simulink model "sampleModel1488"  (R2023a)
settings: Solver=VariableStepAuto  StartTime=0.0  StopTime=10.0  RelTol=1e-3
undefined symbols (not defined in the file): b011101a, b0c8, bf87616c, DiscIntNeverNeededParam, Newton, Raphson
libraries: simulink x171, slpidlib x32, simulink_need_slupdate x2
(part 1 of 6)
settings Model: Creator=TSMC  LastModifiedBy=TSMC

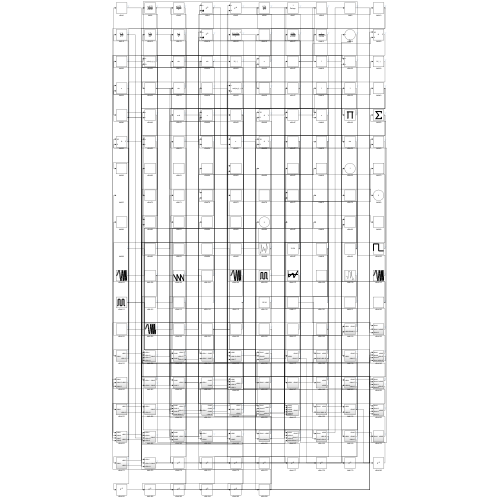
[thumbnail: Simulink's stored preview of the top-level diagram]
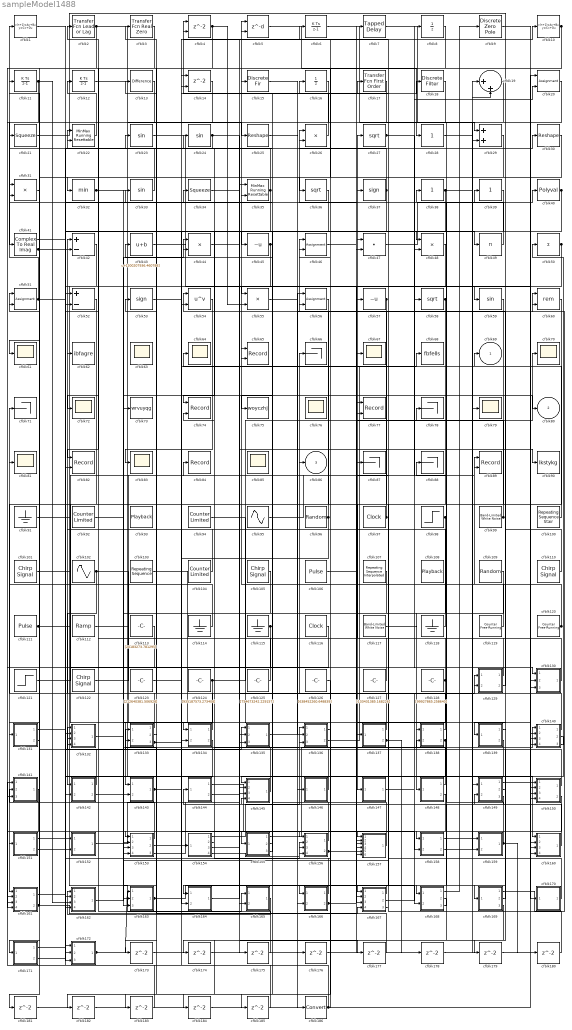
== system sampleModel1488 ==
  cfblk1 : DiscreteStateSpace
  cfblk10 : DiscreteStateSpace
  cfblk100 : simulink/Sources/Repeating Sequence Stair  OutValues=[-762369518.443559, -847374089.038324]  tsamp=-1  OutMin=[]  OutMax=[]  OutDataTypeStr=double  OutputDataTypeScalingMode=double  OutDataType=fixdt(0,8)  ConRadixGroup=Best Precision: Vector-wise  OutScaling=2^-12
  cfblk101 : simulink/Sources/Chirp Signal  f1=[899816213.693097]  T=[-380286117.262630]  f2=[198637424.557367]
  cfblk102 : Sin  Amplitude=[-477515735.570016]  Bias=[72041173.991796]  SampleTime=0
  cfblk103 : simulink/Sources/Repeating Sequence  rep_seq_t=[0 2]  rep_seq_y=[-391359167.323341, -994559578.240211]
  cfblk104 : simulink/Sources/Counter Limited  uplimit=[518.000000]  tsamp=-1
  cfblk105 : simulink/Sources/Chirp Signal  f1=[828543943.259845]  T=[-687971089.943261]  f2=[529515713.712588]
  cfblk106 : DiscretePulseGenerator  PulseType=Time based  Amplitude=[720280650.254154]  Period=[58198645.361039]  PulseWidth=5  PhaseDelay=[7.000000]
  cfblk107 : simulink/Sources/Repeating Sequence Interpolated  OutValues=[129302697.254445, -483455900.765630, 289136432.217906, -604021489.155862, 732674675.731693]  TimeValues=[0 0.1 0.5 0.6 1].'  LookUpMeth=Use Input Below  tsamp=0.01  OutMin=[]  OutMax=[]  OutDataTypeStr=double  OutputDataTypeScalingMode=double  OutDataType=fixdt(0,8)  OutScaling=2^-10
  cfblk108 : Playback  NumPorts=0  PartName=b011101a-6eb5-4819-b0c8-95222edf8c13
  cfblk109 : RandomNumber  Mean=[-63804.166528]  Variance=[5878.142676]  Seed=[575719339.000000]  SampleTime=0.1
  cfblk11 : DiscreteIntegrator  ICPrevOutput=DiscIntNeverNeededParam  ICPrevScaledInput=DiscIntNeverNeededParam
  cfblk110 : simulink/Sources/Chirp Signal  f1=[-302225759.290162]  T=[865618805.379564]  f2=[-592318645.179689]
  cfblk111 : DiscretePulseGenerator  PulseType=Time based  Amplitude=[753444769.039848]  Period=[70377866.971397]  PulseWidth=5  PhaseDelay=[4.000000]
  cfblk112 : simulink/Sources/Ramp  slope=[-695.666721]  start=[46.584433]  InitialOutput=[-395183.012407]
  cfblk113 : Constant  Value=[20183273.781295]  SampleTime=1
  cfblk{91,114..115,118} (4 alike) : Ground
  cfblk116 : DigitalClock
  cfblk117 : simulink/Sources/Band-Limited White Noise  Cov=[1552995708.106671]  Ts=0.1  seed=[2294206463.000000]
  cfblk119 : simulink/Sources/Counter Free-Running  NumBits=[2.000000]  tsamp=-1
  cfblk12 : DiscreteIntegrator  ICPrevOutput=DiscIntNeverNeededParam  ICPrevScaledInput=DiscIntNeverNeededParam
  cfblk120 : simulink/Sources/Counter Free-Running  NumBits=[18.000000]  tsamp=-1
  cfblk121 : Step  Time=[19.000000]  Before=[420474009.001986]  After=[851009496.390192]  SampleTime=0
  cfblk122 : simulink/Sources/Chirp Signal  f1=[-178285749.618264]  T=[-856050795.136190]  f2=[-767698347.330060]
  cfblk123 : Constant  Value=[212640381.506928]  SampleTime=1
  cfblk124 : Constant  Value=[935187573.273408]  SampleTime=1
  cfblk125 : Constant  Value=[754673242.229157]  SampleTime=1
  cfblk126 : Constant  Value=[638452260.648839]  SampleTime=1
  cfblk127 : Constant  Value=[133431385.168226]  SampleTime=1
  cfblk128 : Constant  Value=[99927865.258640]  SampleTime=1
  cfblk129 : Subsystem
  cfblk13 : simulink/Discrete/Difference  ICPrevInput=0.0  OutMin=[]  OutMax=[]  OutDataTypeStr=Inherit: Inherit via back propagation  OutDataType=fixdt(1, 16)  OutScaling=2^-10  DoSatur=off
  cfblk130 : Subsystem
  cfblk131 : Subsystem
  cfblk132 : Subsystem
  cfblk133 : Subsystem
  cfblk134 : Subsystem
  cfblk135 : Subsystem
  cfblk136 : Subsystem
  cfblk137 : Subsystem
  cfblk138 : Subsystem
  cfblk139 : Subsystem
  cfblk14 : Delay  ShowEnablePort=on  SampleTime=1
      settings: InputPortMap=u0,e6
  cfblk140 : Subsystem
  cfblk141 : Subsystem
  cfblk142 : Subsystem
  cfblk143 : Subsystem
  cfblk144 : Subsystem
  cfblk145 : Subsystem
  cfblk146 : Subsystem
  cfblk147 : Subsystem
  cfblk148 : Subsystem
  cfblk149 : Subsystem
  cfblk15 : DiscreteFir  SampleTime=1
  cfblk150 : Subsystem
  cfblk151 : Subsystem
  cfblk152 : Subsystem
  cfblk153 : Subsystem
  cfblk154 : Subsystem
  cfblk155 : Subsystem
  cfblk156 : Subsystem
  cfblk157 : Subsystem
  cfblk158 : Subsystem
  cfblk159 : Subsystem
  cfblk16 : UnitDelay  HasFrameUpgradeWarning=on
  cfblk160 : Subsystem
  cfblk161 : Subsystem
  cfblk162 : Subsystem
  cfblk163 : Subsystem
  cfblk164 : Subsystem
  cfblk165 : Subsystem
  cfblk166 : Subsystem
  cfblk167 : Subsystem
  cfblk168 : Subsystem
  cfblk169 : Subsystem
  cfblk17 : simulink/Discrete/Transfer Fcn First Order  PoleZ=0.95  ICPrevOutput=0.0  DoSatur=off
  cfblk170 : Subsystem
  cfblk171 : Subsystem
  cfblk172 : Subsystem
  cfblk{173..185} (13 alike) : Delay  SampleTime=1
  cfblk18 : DiscreteFilter  SampleTime=1
  cfblk186 : DataTypeConversion  SaturateOnIntegerOverflow=off  RndMeth=Floor
  cfblk19 : Sum  Inputs=|++
  cfblk2 : simulink/Discrete/Transfer Fcn Lead or Lag  PoleZ=0.95  ZeroZ=0.75  ICPrevOutput=0.0  ICPrevInput=0.0  DoSatur=off
  cfblk{20,46,51,56} (4 alike) : Assignment  DiagnosticForDimensions=Warning  IndexOptions=Index vector (dialog)  Indices=1  OutputSizes=1
  cfblk21 : Squeeze
  cfblk22 : simulink/Math Operations/MinMax Running Resettable  Function=min  vinit=0.0
  cfblk{23..24,33,59} (4 alike) : Trigonometry
  cfblk25 : Reshape
  cfblk{26,44,48,55} (4 alike) : Product  Inputs=**
  cfblk27 : Sqrt
  cfblk28 : simulink/Math Operations/Slider Gain  gain=1  low=0  high=2
  cfblk29 : Sum
  cfblk3 : simulink/Discrete/Transfer Fcn Real Zero  ZeroZ=0.75  ICPrevInput=0.0  DoSatur=off
  cfblk30 : Reshape
  cfblk31 : Product
  cfblk32 : MinMax
  cfblk34 : Squeeze
  cfblk35 : simulink/Math Operations/MinMax Running Resettable  Function=min  vinit=0.0
  cfblk36 : Sqrt
  cfblk37 : Signum
  cfblk38 : simulink/Math Operations/Slider Gain  gain=1  low=0  high=2
  cfblk39 : simulink/Math Operations/Slider Gain  gain=1  low=0  high=2
  cfblk4 : Delay  ShowEnablePort=on  SampleTime=1
      settings: InputPortMap=u0,e6
  cfblk40 : Polyval  Coefs=[ +2.081618890e-019, -1.441693666e-014, +4.719686976e-010, -8.536869453e-006, +1.621573104e-001, -8.087801117e+001 ]
  cfblk41 : ComplexToRealImag
  cfblk42 : Sum  Inputs=+-
  cfblk43 : Bias  Bias=[200207936.460788]  SaturateOnIntegerOverflow=off
  cfblk45 : UnaryMinus
  cfblk47 : DotProduct  OutDataTypeStr=Inherit: Inherit via internal rule
  cfblk49 : Product  Inputs=*
  cfblk5 : Delay  DelayLengthSource=Input port  SampleTime=1
      settings: InputPortMap=u0,p1
  cfblk50 : Sum  Inputs=+
  cfblk52 : Sum  Inputs=+-
  cfblk53 : Signum
  cfblk54 : Math  Operator=pow
  cfblk57 : UnaryMinus
  cfblk58 : Sqrt
  cfblk6 : DiscreteIntegrator  ICPrevOutput=DiscIntNeverNeededParam  ICPrevScaledInput=DiscIntNeverNeededParam
  cfblk60 : Math  Operator=rem
  cfblk{61,63..64,67,70,72,76,79,81,83,85} (11 alike) : Scope
      cfblk63 settings: Floating=on
      cfblk76 settings: Floating=on
      cfblk85 settings: Floating=on
  cfblk62 : ToWorkspace  VariableName=ibfagre  SaveFormat=Timeseries  SampleTime=-1
  cfblk65 : Record  FileSettingsInternal="{\"entries\":[{\"content\":{\"excelSettings\":{\"content\":{},\"type\":\"Streamout.ExcelSettings\"}},\"type\":\"Streamout.FileSettingStorage\",\"uuid\":\"\"}],\"packageUris\":[\"http:\\/\\/schema.mathworks.com\\/mf0\\/streamout_blocks\\/R2020a\"],\"version\":\"1.0\"}"  Layout=[1 1]  SignalsInternal="{\"entries\":[{\"content\":{\"signals\":[{\"content\":{\"blockPath\":[],\"dimensions\":[1],\"domain\":\"\",\"lineColor\":\"#a2142f\",\"plots\":[1],\"port\":1,\"sid\":[\"\"],\"signalID\":13705,\"signalName\":\"cfblk143\"},\"type\":\"RecordBlkView.Signal\",\"uuid\":\"\"},{\"content\":{\"blockPath\":[],\"dimensions\":[1],\"domain\":\"\",\"lineColor\":\"#139fff\",\"plots\":[1],\"port\":2,\"sid\":[\"\"],\"signalID\":13793,\"signalName\":\"cfblk115\"},\"type\":\"RecordBlkView.Signal\",\"uuid\":\"\"}]},\"type\":\"RecordBlkView.InputSignals\",\"uuid\":\"\"}],\"packageUris\":[\"http:\\/\\/schema.mathworks.com\\/mf0\\/streamout_blocks\\/R2020a\"],\"version\":\"1.0\"}"  VisualizationBindings="{\"xyplotplugin\":{\"info\":[{\"series\":[{\"bindingParametersList\":[{\"parameter\":\"X-Axis\",\"signalID\":13705,\"signalName\":\"cfblk143\"},{\"parameter\":\"Y-Axis\",\"signalID\":13793,\"signalName\":\"cfblk115\"}],\"seriesID\":56317}],\"subplotID\":1}]}}"  CompatibilityTag=XY
  cfblk{66,71,78,87..88} (5 alike) : Terminator
  cfblk68 : ToWorkspace  VariableName=fbfells  SaveFormat=Timeseries  SampleTime=-1
  cfblk7 : simulink/Discrete/Tapped Delay  vinit=0.0  samptime=-1  NumDelays=1  DelayOrder=Oldest  includeCurrent=off
  cfblk73 : ToWorkspace  VariableName=wrvuyqg  SaveFormat=Timeseries  SampleTime=-1
  cfblk74 : Record  FileSettingsInternal="{\"entries\":[{\"content\":{\"excelSettings\":{\"content\":{},\"type\":\"Streamout.ExcelSettings\"}},\"type\":\"Streamout.FileSettingStorage\",\"uuid\":\"\"}],\"packageUris\":[\"http:\\/\\/schema.mathworks.com\\/mf0\\/streamout_blocks\\/R2020a\"],\"version\":\"1.0\"}"  Layout=[1 1]  SignalsInternal="{\"entries\":[{\"content\":{\"signals\":[{\"content\":{\"blockPath\":[],\"dimensions\":[1],\"domain\":\"\",\"lineColor\":\"#a2142f\",\"plots\":[1],\"port\":1,\"sid\":[\"\"],\"signalID\":13709,\"signalName\":\"cfblk40\"},\"type\":\"RecordBlkView.Signal\",\"uuid\":\"\"},{\"content\":{\"blockPath\":[],\"dimensions\":[1],\"domain\":\"\",\"lineColor\":\"#139fff\",\"plots\":[1],\"port\":2,\"sid\":[\"\"],\"signalID\":13713,\"signalName\":\"cfblk166:1\"},\"type\":\"RecordBlkView.Signal\",\"uuid\":\"\"}]},\"type\":\"RecordBlkView.InputSignals\",\"uuid\":\"\"}],\"packageUris\":[\"http:\\/\\/schema.mathworks.com\\/mf0\\/streamout_blocks\\/R2020a\"],\"version\":\"1.0\"}"  VisualizationBindings="{\"xyplotplugin\":{\"info\":[{\"series\":[{\"bindingParametersList\":[{\"parameter\":\"X-Axis\",\"signalID\":13709,\"signalName\":\"cfblk40\"},{\"parameter\":\"Y-Axis\",\"signalID\":13713,\"signalName\":\"cfblk166:1\"}],\"seriesID\":40022}],\"subplotID\":1}]}}"  CompatibilityTag=XY
  cfblk75 : ToWorkspace  VariableName=woyczhj  SaveFormat=Timeseries  SampleTime=-1
  cfblk77 : Record  FileSettingsInternal="{\"entries\":[{\"content\":{\"excelSettings\":{\"content\":{},\"type\":\"Streamout.ExcelSettings\"}},\"type\":\"Streamout.FileSettingStorage\",\"uuid\":\"\"}],\"packageUris\":[\"http:\\/\\/schema.mathworks.com\\/mf0\\/streamout_blocks\\/R2020a\"],\"version\":\"1.0\"}"  Layout=[1 1]  SignalsInternal="{\"entries\":[{\"content\":{\"signals\":[{\"content\":{\"blockPath\":[],\"dimensions\":[1],\"domain\":\"\",\"lineColor\":\"#a2142f\",\"plots\":[1],\"port\":1,\"sid\":[\"\"],\"signalID\":13773,\"signalName\":\"cfblk99\"},\"type\":\"RecordBlkView.Signal\",\"uuid\":\"\"},{\"content\":{\"blockPath\":[],\"dimensions\":[1],\"domain\":\"\",\"lineColor\":\"#139fff\",\"plots\":[1],\"port\":2,\"sid\":[\"\"],\"signalID\":13777,\"signalName\":\"cfblk99\"},\"type\":\"RecordBlkView.Signal\",\"uuid\":\"\"}]},\"type\":\"RecordBlkView.InputSignals\",\"uuid\":\"\"}],\"packageUris\":[\"http:\\/\\/schema.mathworks.com\\/mf0\\/streamout_blocks\\/R2020a\"],\"version\":\"1.0\"}"  VisualizationBindings="{\"xyplotplugin\":{\"info\":[{\"series\":[{\"bindingParametersList\":[{\"parameter\":\"X-Axis\",\"signalID\":13773,\"signalName\":\"cfblk99\"},{\"parameter\":\"Y-Axis\",\"signalID\":13777,\"signalName\":\"cfblk99\"}],\"seriesID\":53659}],\"subplotID\":1}]}}"  CompatibilityTag=XY
  cfblk8 : UnitDelay  HasFrameUpgradeWarning=on
  cfblk82 : Record  FileSettingsInternal="{\"entries\":[{\"content\":{\"excelSettings\":{\"content\":{},\"type\":\"Streamout.ExcelSettings\"}},\"type\":\"Streamout.FileSettingStorage\",\"uuid\":\"\"}],\"packageUris\":[\"http:\\/\\/schema.mathworks.com\\/mf0\\/streamout_blocks\\/R2020a\"],\"version\":\"1.0\"}"  Layout=[1 1]  SignalsInternal="{\"entries\":[{\"content\":{\"signals\":[{\"content\":{\"blockPath\":[],\"dimensions\":[1],\"domain\":\"\",\"lineColor\":\"#a2142f\",\"plots\":[1],\"port\":1,\"sid\":[\"\"],\"signalID\":13717,\"signalName\":\"cfblk18\"},\"type\":\"RecordBlkView.Signal\",\"uuid\":\"\"},{\"content\":{\"blockPath\":[],\"dimensions\":[1],\"domain\":\"\",\"lineColor\":\"#139fff\",\"plots\":[1],\"port\":2,\"sid\":[\"\"],\"signalID\":13721,\"signalName\":\"cfblk151:2\"},\"type\":\"RecordBlkView.Signal\",\"uuid\":\"\"}]},\"type\":\"RecordBlkView.InputSignals\",\"uuid\":\"\"}],\"packageUris\":[\"http:\\/\\/schema.mathworks.com\\/mf0\\/streamout_blocks\\/R2020a\"],\"version\":\"1.0\"}"  VisualizationBindings="{\"xyplotplugin\":{\"info\":[{\"series\":[{\"bindingParametersList\":[{\"parameter\":\"X-Axis\",\"signalID\":13717,\"signalName\":\"cfblk18\"},{\"parameter\":\"Y-Axis\",\"signalID\":13721,\"signalName\":\"cfblk151:2\"}],\"seriesID\":20221}],\"subplotID\":1}]}}"  CompatibilityTag=XY
  cfblk84 : Record  FileSettingsInternal="{\"entries\":[{\"content\":{\"excelSettings\":{\"content\":{},\"type\":\"Streamout.ExcelSettings\"}},\"type\":\"Streamout.FileSettingStorage\",\"uuid\":\"\"}],\"packageUris\":[\"http:\\/\\/schema.mathworks.com\\/mf0\\/streamout_blocks\\/R2020a\"],\"version\":\"1.0\"}"  SignalsInternal="{\"entries\":[{\"content\":{\"signals\":[{\"content\":{\"blockPath\":[],\"dimensions\":[1],\"domain\":\"\",\"lineColor\":\"#d95319\",\"plots\":[1],\"port\":1,\"sid\":[\"\"],\"signalID\":13697,\"signalName\":\"cfblk142:2\"},\"type\":\"RecordBlkView.Signal\",\"uuid\":\"\"}]},\"type\":\"RecordBlkView.InputSignals\",\"uuid\":\"\"}],\"packageUris\":[\"http:\\/\\/schema.mathworks.com\\/mf0\\/streamout_blocks\\/R2020a\"],\"version\":\"1.0\"}"  VisualizationBindings="{\"sparklinesplugin\":{\"info\":[{\"bindingParametersList\":[],\"subplotID\":1}]}}"
  cfblk89 : Record  FileSettingsInternal="{\"entries\":[{\"content\":{\"excelSettings\":{\"content\":{},\"type\":\"Streamout.ExcelSettings\"}},\"type\":\"Streamout.FileSettingStorage\",\"uuid\":\"\"}],\"packageUris\":[\"http:\\/\\/schema.mathworks.com\\/mf0\\/streamout_blocks\\/R2020a\"],\"version\":\"1.0\"}"  Layout=[1 1]  SignalsInternal="{\"entries\":[{\"content\":{\"signals\":[{\"content\":{\"blockPath\":[],\"dimensions\":[1],\"domain\":\"\",\"lineColor\":\"#a2142f\",\"plots\":[1],\"port\":1,\"sid\":[\"\"],\"signalID\":13725,\"signalName\":\"cfblk156:2\"},\"type\":\"RecordBlkView.Signal\",\"uuid\":\"\"},{\"content\":{\"blockPath\":[],\"dimensions\":[1],\"domain\":\"\",\"lineColor\":\"#139fff\",\"plots\":[1],\"port\":2,\"sid\":[\"\"],\"signalID\":13729,\"signalName\":\"cfblk120\"},\"type\":\"RecordBlkView.Signal\",\"uuid\":\"\"}]},\"type\":\"RecordBlkView.InputSignals\",\"uuid\":\"\"}],\"packageUris\":[\"http:\\/\\/schema.mathworks.com\\/mf0\\/streamout_blocks\\/R2020a\"],\"version\":\"1.0\"}"  VisualizationBindings="{\"xyplotplugin\":{\"info\":[{\"series\":[{\"bindingParametersList\":[{\"parameter\":\"X-Axis\",\"signalID\":13725,\"signalName\":\"cfblk156:2\"},{\"parameter\":\"Y-Axis\",\"signalID\":13729,\"signalName\":\"cfblk120\"}],\"seriesID\":42703}],\"subplotID\":1}]}}"  CompatibilityTag=XY
  cfblk9 : DiscreteZeroPole  Poles=[0 0.5]  Gain=1
  cfblk90 : ToWorkspace  VariableName=lkstykg  SaveFormat=Timeseries  SampleTime=-1
  cfblk92 : simulink/Sources/Counter Limited  uplimit=[326.000000]  tsamp=-1
  cfblk93 : Playback  NumPorts=0  PartName=bf87616c-5d9a-425c-8382-97f2101e7582
  cfblk94 : simulink/Sources/Counter Limited  uplimit=[272.000000]  tsamp=-1
  cfblk95 : Sin  Amplitude=[644063288.988140]  Bias=[-805736722.000747]  SampleTime=0
  cfblk96 : UniformRandomNumber  Minimum=[-3474527164.440428]  Maximum=[5792684049.371810]  Seed=[15645962.000000]  SampleTime=0.1
  cfblk97 : DigitalClock
  cfblk98 : Step  Time=[14.000000]  Before=[644954690.237287]  After=[-26029377.976469]  SampleTime=0
  cfblk99 : simulink/Sources/Band-Limited White Noise  Cov=[1766860614.703701]  Ts=0.1  seed=[5558870258.000000]
  cfblk69 : Outport
  cfblk80 : Outport  Port=2
  cfblk86 : Outport  Port=3
  wires:
  cfblk168/1(cfblk2) -> cfblk9/1
  cfblk109/1 -> cfblk148/1(cfblk1)
  cfblk26/1 -> cfblk4/1
  cfblk163/1(cfblk2) -> cfblk166/1(cfblk1), cfblk18/1
  cfblk112/1 -> cfblk66/1
  cfblk52/1 -> cfblk134/1(cfblk1)
  cfblk144/1(cfblk2) -> cfblk157/1(cfblk1)
  cfblk21/1 -> cfblk139/1(cfblk1)
  cfblk3/1 -> cfblk165/1(cfblk1)
  cfblk5/1 -> cfblk28/1
  cfblk111/1 -> cfblk143/1(cfblk1), cfblk167/2(cfblk13)
  cfblk2/1 -> cfblk160/1(cfblk1), cfblk131/1(cfblk1)
  cfblk120/1 -> cfblk5/1, cfblk89/2
  cfblk49/1 -> cfblk26/1
  cfblk38/1 -> cfblk159/1(cfblk1), cfblk162/4(cfblk11)
  cfblk130/1(cfblk2) -> cfblk26/2
  cfblk107/1 -> cfblk166/2(cfblk12)
  cfblk114/1 -> cfblk71/1
  cfblk32/1 -> cfblk45/1, cfblk80/1
  cfblk147/1(cfblk2) -> cfblk140/1(cfblk1)
  cfblk33/1 -> cfblk23/1
  cfblk154/1(cfblk2) -> cfblk136/1(cfblk1)
  cfblk170/1(cfblk2) -> cfblk16/1
  cfblk150/1(cfblk2) -> cfblk133/1(cfblk1)
  cfblk148/1(cfblk2) -> cfblk54/1
  cfblk53/1 -> cfblk5/2
  cfblk36/1 -> cfblk134/2(cfblk6)
  cfblk155/1(cfblk2) -> cfblk20/1
  cfblk58/1 -> cfblk147/1(cfblk1), cfblk167/1(cfblk1)
  cfblk141/1(cfblk2) -> cfblk161/1(cfblk1)
  cfblk51/1 -> cfblk1/1, cfblk34/1
  cfblk168/3(cfblk11) -> cfblk144/1(cfblk1)
  cfblk104/1 -> cfblk42/1
  cfblk54/1 -> cfblk83/1
  cfblk57/1 -> cfblk151/1(cfblk1), cfblk157/5(cfblk10)
  cfblk142/1(cfblk2) -> cfblk51/1
  cfblk155/2(cfblk7) -> cfblk33/1
  cfblk23/1 -> cfblk59/1
  cfblk17/1 -> cfblk41/1
  cfblk143/1(cfblk2) -> cfblk65/1, cfblk157/3(cfblk8)
  cfblk96/1 -> cfblk46/1, cfblk164/2(cfblk8)
  cfblk12/1 -> cfblk25/1
  cfblk137/1(cfblk2) -> cfblk53/1
  cfblk160/1(cfblk2) -> cfblk149/2(cfblk14)
  cfblk106/1 -> cfblk27/1
  cfblk47/1 -> cfblk39/1
  cfblk134/1(cfblk2) -> cfblk81/1
  cfblk6/1 -> cfblk29/1
  cfblk19/1 -> cfblk168/1(cfblk1)
  cfblk125/1 -> cfblk13/1
  cfblk119/1 -> cfblk15/1
  cfblk13/1 -> cfblk61/1
  cfblk164/1(cfblk2) -> cfblk37/1
  cfblk39/1 -> cfblk136/2(cfblk10)
  cfblk4/1 -> cfblk52/2, cfblk55/2
  cfblk118/1 -> cfblk2/1
  cfblk7/1 -> cfblk79/1
  cfblk102/1 -> cfblk142/1(cfblk1), cfblk154/1(cfblk1)
  cfblk145/1(cfblk2) -> cfblk24/1
  cfblk156/1(cfblk2) -> cfblk43/1
  cfblk165/1(cfblk2) -> cfblk162/1(cfblk1)
  cfblk10/1 -> cfblk36/1, cfblk161/4(cfblk8)
  cfblk97/1 -> cfblk47/1, cfblk44/2
  cfblk131/1(cfblk2) -> cfblk172/1(cfblk1)
  cfblk140/1(cfblk2) -> cfblk17/1
  cfblk134/2(cfblk7) -> cfblk142/2(cfblk8)
  cfblk137/2(cfblk16) -> cfblk4/2, cfblk178/1
  cfblk153/1(cfblk2) -> cfblk141/2(cfblk12)
  cfblk11/1 -> cfblk141/3(cfblk13), cfblk162/3(cfblk10)
  cfblk91/1 -> cfblk130/1(cfblk1)
  cfblk161/1(cfblk2) -> cfblk135/1(cfblk1)
  cfblk159/1(cfblk2) -> cfblk88/1, cfblk180/1
  cfblk100/1 -> cfblk64/1
  cfblk142/2(cfblk9) -> cfblk84/1
  cfblk138/1(cfblk2) -> cfblk86/1
  cfblk140/2(cfblk12) -> cfblk145/1(cfblk1)
  cfblk146/1(cfblk2) -> cfblk132/1(cfblk1)
  cfblk169/1(cfblk2) -> cfblk60/1
  cfblk155/3(cfblk8) -> cfblk21/1
  cfblk150/2(cfblk13) -> cfblk169/1(cfblk1)
  cfblk116/1 -> cfblk135/2(cfblk16)
  cfblk129/1(cfblk2) -> cfblk78/1
  cfblk131/2(cfblk11) -> cfblk51/2
  cfblk98/1 -> cfblk143/2(cfblk11), cfblk157/6(cfblk11)
  cfblk124/1 -> cfblk70/1, cfblk160/4(cfblk14), cfblk153/3(cfblk14)
  cfblk128/1 -> cfblk22/1, cfblk157/2(cfblk7)
  cfblk27/1 -> cfblk130/2(cfblk11), cfblk20/2
  cfblk92/1 -> cfblk73/1
  cfblk172/1(cfblk2) -> cfblk163/1(cfblk1), cfblk57/1
  cfblk110/1 -> cfblk69/1
  cfblk133/1(cfblk2) -> cfblk62/1
  cfblk135/1(cfblk2) -> cfblk60/2
  cfblk121/1 -> cfblk58/1
  cfblk139/1(cfblk2) -> cfblk158/1(cfblk1)
  cfblk50/1 -> cfblk75/1, cfblk167/3(cfblk14)
  cfblk152/1(cfblk2) -> cfblk68/1
  cfblk127/1 -> cfblk67/1
  cfblk101/1 -> cfblk56/1
  cfblk136/2(cfblk12) -> cfblk8/1
  cfblk156/2(cfblk16) -> cfblk89/1, cfblk138/2(cfblk9)
  cfblk30/1 -> cfblk135/3(cfblk17)
  cfblk18/1 -> cfblk82/1
  cfblk153/2(cfblk16) -> cfblk10/1
  cfblk105/1 -> cfblk145/2(cfblk9)
  cfblk162/1(cfblk2) -> cfblk136/3(cfblk11)
  cfblk158/1(cfblk2) -> cfblk40/1
  cfblk117/1 -> cfblk138/1(cfblk1)
  cfblk103/1 -> cfblk146/1(cfblk1)
  cfblk14/1 -> cfblk32/1
  cfblk149/1(cfblk2) -> cfblk140/3(cfblk10)
  cfblk148/2(cfblk9) -> cfblk161/2(cfblk6)
  cfblk48/1 -> cfblk54/2
  cfblk138/2(cfblk10) -> cfblk38/1, cfblk157/4(cfblk9)
  cfblk171/1(cfblk2) -> cfblk42/2
  cfblk44/1 -> cfblk145/3(cfblk10)
  cfblk29/1 -> cfblk171/1(cfblk1)
  cfblk99/1 -> cfblk77/1, cfblk77/2
  cfblk15/1 -> cfblk168/2(cfblk9)
  cfblk115/1 -> cfblk65/2, cfblk161/3(cfblk7)
  cfblk140/3(cfblk13) -> cfblk50/1
  cfblk35/1 -> cfblk3/1, cfblk163/3(cfblk9)
  cfblk158/2(cfblk14) -> cfblk29/2
  cfblk123/1 -> cfblk14/2
  cfblk28/1 -> cfblk19/2
  cfblk42/1 -> cfblk172/2(cfblk13)
  cfblk25/1 -> cfblk49/1
  cfblk153/3(cfblk17) -> cfblk129/1(cfblk1)
  cfblk94/1 -> cfblk186/1
  cfblk95/1 -> cfblk7/1
  cfblk167/1(cfblk2) -> cfblk165/2(cfblk9)
  cfblk122/1 -> cfblk47/2
  cfblk43/1 -> cfblk130/3(cfblk12)
  cfblk167/2(cfblk16) -> cfblk129/2(cfblk10)
  cfblk167/3(cfblk17) -> cfblk87/1
  cfblk45/1 -> cfblk72/1, cfblk155/1(cfblk1)
  cfblk126/1 -> cfblk156/1(cfblk1)
  cfblk20/1 -> cfblk132/2(cfblk12)
  cfblk169/2(cfblk9) -> cfblk132/3(cfblk13)
  cfblk41/1 -> cfblk150/3(cfblk11)
  cfblk59/1 -> cfblk172/3(cfblk14)
  cfblk133/2(cfblk15) -> cfblk163/2(cfblk8)
  cfblk60/1 -> cfblk159/2(cfblk12)
  cfblk149/2(cfblk15) -> cfblk164/1(cfblk1)
  cfblk24/1 -> cfblk90/1, cfblk22/2
  cfblk161/2(cfblk9) -> cfblk31/1, cfblk167/4(cfblk15)
  cfblk46/1 -> cfblk48/1
  cfblk171/2(cfblk8) -> cfblk156/2(cfblk13)
  cfblk133/3(cfblk16) -> cfblk158/2(cfblk13), cfblk153/1(cfblk1)
  cfblk40/1 -> cfblk74/1, cfblk153/4(cfblk15), cfblk179/1
  cfblk56/1 -> cfblk162/2(cfblk9)
  cfblk166/1(cfblk2) -> cfblk74/2
  cfblk157/1(cfblk2) -> cfblk132/4(cfblk14)
  cfblk22/1 -> cfblk12/1
  cfblk129/2(cfblk11) -> cfblk56/2
  cfblk41/2 -> cfblk150/4(cfblk12), cfblk11/1, cfblk35/2
  cfblk151/1(cfblk2) -> cfblk30/1
  cfblk9/1 -> cfblk170/1(cfblk1)
  cfblk37/1 -> cfblk6/1, cfblk55/1
  cfblk154/2(cfblk8) -> cfblk31/2
  cfblk113/1 -> cfblk152/2(cfblk16)
  cfblk132/1(cfblk2) -> cfblk44/1
  cfblk1/1 -> cfblk48/2
  cfblk149/3(cfblk16) -> cfblk145/4(cfblk11)
  cfblk151/2(cfblk16) -> cfblk82/2
  cfblk166/2(cfblk13) -> cfblk137/1(cfblk1), cfblk46/2
  cfblk154/3(cfblk9) -> cfblk35/1
  cfblk154/4(cfblk10) -> cfblk156/3(cfblk14)
  cfblk16/1 -> cfblk173/1
  cfblk173/1 -> cfblk140/2(cfblk9)
  cfblk168/2(cfblk10) -> cfblk174/1
  cfblk174/1 -> cfblk19/1
  cfblk34/1 -> cfblk175/1
  cfblk175/1 -> cfblk52/1
  cfblk55/1 -> cfblk176/1
  cfblk176/1 -> cfblk149/1(cfblk1)
  cfblk144/2(cfblk8) -> cfblk177/1
  cfblk177/1 -> cfblk133/2(cfblk14)
  cfblk178/1 -> cfblk160/2(cfblk12)
  cfblk179/1 -> cfblk160/3(cfblk13)
  cfblk180/1 -> cfblk153/2(cfblk13)
  cfblk31/1 -> cfblk181/1
  cfblk181/1 -> cfblk150/1(cfblk1)
  cfblk136/1(cfblk2) -> cfblk182/1
  cfblk182/1 -> cfblk150/2(cfblk10)
  cfblk8/1 -> cfblk183/1
  cfblk183/1 -> cfblk141/1(cfblk1)
  cfblk169/3(cfblk10) -> cfblk184/1
  cfblk184/1 -> cfblk140/4(cfblk11)
  cfblk139/2(cfblk13) -> cfblk185/1
  cfblk185/1 -> cfblk14/1
  cfblk186/1 -> cfblk156/4(cfblk15), cfblk152/1(cfblk1)

== system sampleModel1488/cfblk129 ==
  cfblk1 : Inport
  cfblk10 : Inport  Port=2
  cfblk12 : Delay  SampleTime=1
  cfblk13 : Delay  SampleTime=1
  cfblk3 : DiscreteFir  SampleTime=1
  cfblk4 : Signum
  cfblk5 : Assignment  DiagnosticForDimensions=Warning  IndexOptions=Index vector (dialog)  Indices=1  OutputSizes=1
  cfblk6 : Polyval  Coefs=[ +2.081618890e-019, -1.441693666e-014, +4.719686976e-010, -8.536869453e-006, +1.621573104e-001, -8.087801117e+001 ]
  cfblk7 : Subsystem
  cfblk8 : Subsystem
  cfblk9 : Subsystem
  cfblk2 : Outport
  cfblk11 : Outport  Port=2
  wires:
  cfblk5/1 -> cfblk2/1, cfblk7/2(cfblk14)
  cfblk8/1(cfblk2) -> cfblk11/1
  cfblk4/1 -> cfblk5/1
  cfblk3/1 -> cfblk6/1, cfblk13/1
  cfblk7/1(cfblk2) -> cfblk3/1, cfblk8/3(cfblk9)
  cfblk1/1 -> cfblk9/1(cfblk1), cfblk5/2
  cfblk9/1(cfblk2) -> cfblk8/1(cfblk1), cfblk4/1, cfblk7/3(cfblk15)
  cfblk6/1 -> cfblk8/2(cfblk8), cfblk12/1
  cfblk10/1 -> cfblk9/3(cfblk7)
  cfblk12/1 -> cfblk9/2(cfblk6)
  cfblk13/1 -> cfblk7/1(cfblk1)

== system sampleModel1488/cfblk130 ==
  cfblk1 : Inport
  cfblk11 : Inport  Port=2
  cfblk12 : Inport  Port=3
  cfblk10 : Subsystem
  cfblk{13..17} (5 alike) : Delay  SampleTime=1
  cfblk3 : UnitDelay  HasFrameUpgradeWarning=on
  cfblk4 : Sum  Inputs=+-
  cfblk5 : Trigonometry
  cfblk6 : MinMax  Inputs=3
  cfblk7 : Subsystem
  cfblk8 : Subsystem
  cfblk9 : Subsystem
  cfblk2 : Outport
  wires:
  cfblk12/1 -> cfblk2/1, cfblk10/3(cfblk9)
  cfblk11/1 -> cfblk6/1
  cfblk1/1 -> cfblk3/1, cfblk7/1(cfblk1)
  cfblk10/1(cfblk2) -> cfblk7/3(cfblk11), cfblk14/1
  cfblk3/1 -> cfblk4/2, cfblk10/4(cfblk10), cfblk7/2(cfblk10)
  cfblk4/1 -> cfblk9/2(cfblk12), cfblk7/4(cfblk12)
  cfblk8/1(cfblk2) -> cfblk10/1(cfblk1)
  cfblk9/1(cfblk2) -> cfblk5/1
  cfblk6/1 -> cfblk16/1, cfblk17/1
  cfblk9/2(cfblk14) -> cfblk8/2(cfblk10)
  cfblk7/2(cfblk13) -> cfblk6/2, cfblk6/3
  cfblk9/3(cfblk15) -> cfblk8/3(cfblk11)
  cfblk5/1 -> cfblk13/1
  cfblk13/1 -> cfblk9/1(cfblk1)
  cfblk14/1 -> cfblk4/1
  cfblk7/1(cfblk2) -> cfblk15/1
  cfblk15/1 -> cfblk10/2(cfblk8)
  cfblk16/1 -> cfblk8/1(cfblk1)
  cfblk17/1 -> cfblk9/3(cfblk13)

== system sampleModel1488/cfblk131 ==
  cfblk1 : Inport
  cfblk10 : If  IfExpression=u1 >= 0  SampleTime=1
  cfblk12 : Subsystem  TreatAsAtomicUnit=on
  cfblk13 : Subsystem  TreatAsAtomicUnit=on
  cfblk{14..18} (5 alike) : Delay  SampleTime=1
  cfblk3 : simulink/Discrete/Tapped Delay  vinit=0.0  samptime=-1  NumDelays=1  DelayOrder=Oldest  includeCurrent=off
  cfblk4 : Delay  DelayLengthSource=Input port  SampleTime=1
      settings: InputPortMap=u0,p1
  cfblk5 : Trigonometry
  cfblk6 : UnaryMinus
  cfblk7 : Constant  Value=[-879711208.618790]  SampleTime=1
  cfblk8 : Subsystem
  cfblk9 : Subsystem
  cfblk2 : Outport
  cfblk11 : Outport  Port=2
  wires:
  cfblk6/1 -> cfblk4/1
  cfblk3/1 -> cfblk5/1
  cfblk12/1(cfblk2) -> cfblk8/1(cfblk1)
  cfblk12/2(cfblk6) -> cfblk9/1(cfblk1)
  cfblk8/1(cfblk2) -> cfblk14/1, cfblk17/1
  cfblk1/1 -> cfblk12/1(cfblk1)
  cfblk12/3(cfblk7) -> cfblk3/1
  cfblk9/1(cfblk2) -> cfblk11/1
  cfblk12/4(cfblk8) -> cfblk2/1
  cfblk7/1 -> cfblk6/1
  cfblk13/2(cfblk11) -> cfblk4/2
  cfblk10/1 -> cfblk12/Action
  cfblk10/2 -> cfblk13/Action
  cfblk14/1 -> cfblk10/1
  cfblk13/1(cfblk2) -> cfblk15/1
  cfblk15/1 -> cfblk8/2(cfblk16)
  cfblk4/1 -> cfblk16/1
  cfblk16/1 -> cfblk13/2(cfblk9)
  cfblk17/1 -> cfblk13/3(cfblk10)
  cfblk5/1 -> cfblk18/1
  cfblk18/1 -> cfblk13/1(cfblk1)

== system sampleModel1488/cfblk132 ==
  cfblk1 : Inport
  cfblk12 : Inport  Port=2
  cfblk13 : Inport  Port=3
  cfblk14 : Inport  Port=4
  cfblk10 : Subsystem
  cfblk11 : Subsystem
  cfblk15 : Delay  SampleTime=1
  cfblk16 : Delay  SampleTime=1
  cfblk3 : ComplexToMagnitudeAngle
  cfblk4 : Product  Inputs=*
  cfblk5 : Sqrt  Operator=rSqrt  AlgorithmType=Newton-Raphson
  cfblk6 : Squeeze
  cfblk7 : MinMax
  cfblk8 : Constant  Value=[291262025.743041]  SampleTime=1
  cfblk9 : Subsystem
  cfblk2 : Outport
  wires:
  cfblk9/1(cfblk2) -> cfblk5/1, cfblk2/1, cfblk10/5(cfblk11), cfblk16/1
  cfblk3/1 -> cfblk10/1(cfblk1)
  cfblk5/1 -> cfblk10/2(cfblk8)
  cfblk4/1 -> cfblk11/1(cfblk1)
  cfblk3/2 -> cfblk6/1
  cfblk8/1 -> cfblk7/1
  cfblk6/1 -> cfblk4/1
  cfblk14/1 -> cfblk3/1
  cfblk12/1 -> cfblk9/2(cfblk9)
  cfblk7/1 -> cfblk9/3(cfblk10), cfblk11/3(cfblk13)
  cfblk13/1 -> cfblk10/3(cfblk9)
  cfblk1/1 -> cfblk11/2(cfblk12)
  cfblk11/1(cfblk2) -> cfblk9/4(cfblk11)
  cfblk11/2(cfblk15) -> cfblk10/4(cfblk10)
  cfblk10/1(cfblk2) -> cfblk15/1
  cfblk15/1 -> cfblk9/1(cfblk1)
  cfblk16/1 -> cfblk11/4(cfblk14)

== system sampleModel1488/cfblk133 ==
  cfblk1 : Inport
  cfblk14 : Inport  Port=2
  cfblk10 : Sum  Inputs=+-
  cfblk11 : Subsystem
  cfblk12 : Subsystem
  cfblk13 : Subsystem
  cfblk17 : Delay  SampleTime=1
  cfblk3 : simulink/Discrete/Transfer Fcn Lead or Lag  PoleZ=0.95  ZeroZ=0.75  ICPrevOutput=0.0  ICPrevInput=0.0  DoSatur=off
  cfblk4 : UnitDelay  HasFrameUpgradeWarning=on
  cfblk5 : Signum
  cfblk6 : PermuteDimensions
  cfblk7 : DotProduct  OutDataTypeStr=Inherit: Inherit via internal rule
  cfblk8 : Reshape
  cfblk9 : Sum  Inputs=+-
  cfblk2 : Outport
  cfblk15 : Outport  Port=2
  cfblk16 : Outport  Port=3
  wires:
  cfblk5/1 -> cfblk6/1
  cfblk13/1(cfblk2) -> cfblk2/1
  cfblk10/1 -> cfblk8/1
  cfblk8/1 -> cfblk13/1(cfblk1)
  cfblk9/1 -> cfblk4/1
  cfblk7/1 -> cfblk10/1
  cfblk4/1 -> cfblk7/1
  cfblk3/1 -> cfblk11/1(cfblk1)
  cfblk14/1 -> cfblk16/1
  cfblk6/1 -> cfblk9/2, cfblk17/1
  cfblk11/1(cfblk2) -> cfblk13/2(cfblk8)
  cfblk12/1(cfblk2) -> cfblk7/2
  cfblk12/2(cfblk9) -> cfblk10/2
  cfblk12/3(cfblk10) -> cfblk5/1
  cfblk1/1 -> cfblk15/1
  cfblk11/2(cfblk7) -> cfblk9/1, cfblk12/1(cfblk1)
  cfblk17/1 -> cfblk3/1

== system sampleModel1488/cfblk134 ==
  cfblk1 : Inport
  cfblk6 : Inport  Port=2
  cfblk{10..13} (4 alike) : Delay  SampleTime=1
  cfblk3 : Sum  Inputs=|++
  cfblk4 : Subsystem
  cfblk5 : If  IfExpression=u1 >= 0  SampleTime=1
  cfblk8 : Subsystem  TreatAsAtomicUnit=on
  cfblk9 : Subsystem  TreatAsAtomicUnit=on
  cfblk2 : Outport
  cfblk7 : Outport  Port=2
  wires:
  cfblk3/1 -> cfblk7/1
  cfblk6/1 -> cfblk4/1(cfblk1)
  cfblk9/1(cfblk2) -> cfblk8/1(cfblk1)
  cfblk1/1 -> cfblk9/1(cfblk1)
  cfblk4/1(cfblk2) -> cfblk12/1, cfblk13/1
  cfblk9/2(cfblk13) -> cfblk4/2(cfblk7)
  cfblk9/3(cfblk14) -> cfblk8/2(cfblk6)
  cfblk9/4(cfblk15) -> cfblk3/1
  cfblk9/5(cfblk16) -> cfblk3/2, cfblk4/3(cfblk8), cfblk2/1
  cfblk5/1 -> cfblk8/Action
  cfblk5/2 -> cfblk9/Action
  cfblk8/1(cfblk2) -> cfblk10/1
  cfblk10/1 -> cfblk9/3(cfblk11)
  cfblk8/2(cfblk7) -> cfblk11/1
  cfblk11/1 -> cfblk5/1
  cfblk12/1 -> cfblk9/2(cfblk10)
  cfblk13/1 -> cfblk9/4(cfblk12)

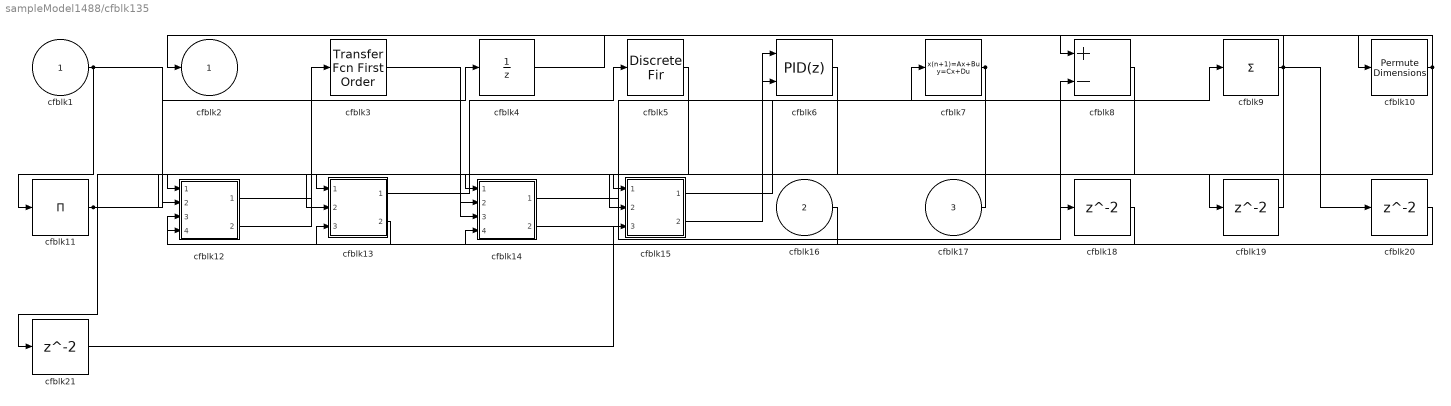
== system sampleModel1488/cfblk135 ==
  cfblk1 : Inport
  cfblk16 : Inport  Port=2
  cfblk17 : Inport  Port=3
  cfblk10 : PermuteDimensions
  cfblk11 : Product  Inputs=*
  cfblk12 : Subsystem
  cfblk13 : Subsystem
  cfblk14 : Subsystem
  cfblk15 : Subsystem
  cfblk{18..21} (4 alike) : Delay  SampleTime=1
  cfblk3 : simulink/Discrete/Transfer Fcn First Order  PoleZ=0.95  ICPrevOutput=0.0  DoSatur=off
  cfblk4 : UnitDelay  HasFrameUpgradeWarning=on
  cfblk5 : DiscreteFir  SampleTime=1
  cfblk6 : slpidlib/PID Controller (2DOF)  Controller=PID  Form=Parallel  TimeDomain=Discrete-time  UseExternalTs=off  SampleTime=1  IntegratorMethod=Forward Euler  FilterMethod=Forward Euler  ControllerParametersSource=internal  P=1  I=1  UseKiTs=off  D=0  N=100  UseFilter=on  b=1  c=1  TunerSelectOption=Transfer Function Based (PID Tuner App)  InitialConditionSource=internal  InitialConditionForIntegrator=0  InitialConditionForFilter=0  DifferentiatorICPrevScaledInput=0  ExternalReset=none  TrackingMode=off  Kt=1  LimitOutput=off  SatLimitsSource=internal  UpperSaturationLimit=inf  LowerSaturationLimit=-inf  LinearizeAsGain=off  AntiWindupMode=none  Kb=1  LimitIntegrator=off  UpperIntegratorSaturationLimit=inf  LowerIntegratorSaturationLimit=-inf  POutMin=[]  POutMax=[]  IOutMin=[]  IOutMax=[]  DOutMin=[]  DOutMax=[]  NOutMin=[]  NOutMax=[]  bOutMin=[]  bOutMax=[]  cOutMin=[]  cOutMax=[]  SumOutMin=[]  SumOutMax=[]  SaturationOutMin=[]  SaturationOutMax=[]  PParamMin=[]  PParamMax=[]  IParamMin=[]  IParamMax=[]  DParamMin=[]  DParamMax=[]  NParamMin=[]  NParamMax=[]  bParamMin=[]  bParamMax=[]  cParamMin=[]  cParamMax=[]  KbParamMin=[]  KbParamMax=[]  KtParamMin=[]  KtParamMax=[]  KbOutMin=[]  KbOutMax=[]  KtOutMin=[]  KtOutMax=[]  IntegratorOutMin=[]  IntegratorOutMax=[]  FilterOutMin=[]  FilterOutMax=[]  SumI1OutMin=[]  SumI1OutMax=[]  SumI2OutMin=[]  SumI2OutMax=[]  SumI3OutMin=[]  SumI3OutMax=[]  SumI4OutMin=[]  SumI4OutMax=[]  SumDOutMin=[]  SumDOutMax=[]  Sum1OutMin=[]  Sum1OutMax=[]  Sum2OutMin=[]  Sum2OutMax=[]  Sum3OutMin=[]  Sum3OutMax=[]  DifferentiatorOutMin=[]  DifferentiatorOutMax=[]  FilterDiffOutCoefMin=[]  FilterDiffOutCoefMax=[]  ReciprocalOutMin=[]  ReciprocalOutMax=[]  SumDenOutMin=[]  SumDenOutMax=[]  SumNumOutMin=[]  SumNumOutMax=[]  DivideOutMin=[]  DivideOutMax=[]  UdiffTsProdOutMin=[]  UdiffTsProdOutMax=[]  NTsProdOutMin=[]  NTsProdOutMax=[]  UintegralTsProdOutMin=[]  UintegralTsProdOutMax=[]  UngainTsProdOutMin=[]  UngainTsProdOutMax=[]  ClampingZeroOutDataTypeStr=Inherit: Inherit via back propagation  ClampingZeroOutMin=[]  ClampingZeroOutMax=[]  FilterDenConstantOutDataTypeStr=Inherit: Inherit via back propagation  FilterDenConstantOutMin=[]  FilterDenConstantOutMax=[]  PCopyOutDataTypeStr=Inherit: Inherit via back propagation  PCopyOutMin=[]  PCopyOutMax=[]  NCopyOutDataTypeStr=Inherit: Inherit via back propagation  NCopyOutMin=[]  NCopyOutMax=[]  IntegratorContinuousStateAttributes=''  IntegratorStateMustResolveToSignalObject=off  IntegratorRTWStateStorageClass=Auto  FilterContinuousStateAttributes=''  FilterStateMustResolveToSignalObject=off  FilterRTWStateStorageClass=Auto  ParallelPVariant=InternalParameters  IdealPVariant=Disabled  IVariant=InternalParameters  DVariant=InternalParameters  bVariant=InternalParameters  cVariant=InternalParameters  IntegratorVariant=Discrete  SatVariant=Disabled  AWVariant=Passthrough  PCopyVariant=Disabled  TRVariant=Disabled  FdbkBlocksVariant=Forward  IdealPFdbkVariant=Disabled  SatFdbkVariant=Disabled  DerivativeFilterVariant=ForwardEulerFilter  NVariant=InternalParameters  NCopyVariant=Disabled  FilterICVariant=InternalICsFilter  IntegratorICVariant=InternalICs  ExternalResetVariant=Disabled  TRSumVariant=Passthrough  SumFdbkVariant=Disabled  SumVariant=Sum_PID  TsampFilterVariant=InternalTs  TsampNgainVariant=Passthrough  TsampIntegralVariant=Disabled_SignalSpec  ExternalSaturationOutDataTypeStr=Inherit: Same as second input
      settings: LibrarySourceBlock=simulink/Discrete/Discrete PID Controller (2DOF)
  cfblk7 : DiscreteStateSpace
  cfblk8 : Sum  Inputs=+-
  cfblk9 : Sum  Inputs=+
  cfblk2 : Outport
  wires:
  cfblk17/1 -> cfblk13/1(cfblk1)
  cfblk13/1(cfblk2) -> cfblk5/1
  cfblk4/1 -> cfblk10/1
  cfblk9/1 -> cfblk2/1, cfblk19/1, cfblk20/1
  cfblk1/1 -> cfblk11/1, cfblk15/1(cfblk1)
  cfblk7/1 -> cfblk6/1, cfblk21/1
  cfblk10/1 -> cfblk8/1, cfblk15/2(cfblk14)
  cfblk11/1 -> cfblk13/2(cfblk6), cfblk4/1
  cfblk15/1(cfblk2) -> cfblk7/1
  cfblk15/2(cfblk16) -> cfblk6/2
  cfblk14/1(cfblk2) -> cfblk8/2
  cfblk5/1 -> cfblk12/2(cfblk7)
  cfblk12/1(cfblk2) -> cfblk14/1(cfblk1)
  cfblk3/1 -> cfblk14/2(cfblk14)
  cfblk16/1 -> cfblk12/3(cfblk8)
  cfblk14/2(cfblk17) -> cfblk9/1
  cfblk12/2(cfblk10) -> cfblk3/1
  cfblk13/2(cfblk8) -> cfblk12/4(cfblk9)
  cfblk6/1 -> cfblk14/3(cfblk15)
  cfblk8/1 -> cfblk18/1
  cfblk18/1 -> cfblk13/3(cfblk7)
  cfblk19/1 -> cfblk12/1(cfblk1)
  cfblk20/1 -> cfblk14/4(cfblk16)
  cfblk21/1 -> cfblk15/3(cfblk15)

== system sampleModel1488/cfblk136 ==
  cfblk1 : Inport
  cfblk10 : Inport  Port=2
  cfblk11 : Inport  Port=3
  cfblk13 : Delay  SampleTime=1
  cfblk14 : Delay  SampleTime=1
  cfblk3 : simulink/Discrete/Transfer Fcn Lead or Lag  PoleZ=0.95  ZeroZ=0.75  ICPrevOutput=0.0  ICPrevInput=0.0  DoSatur=off
  cfblk4 : DiscreteTransferFcn  SampleTime=1
  cfblk5 : Reshape
  cfblk6 : Sqrt  Operator=rSqrt  AlgorithmType=Newton-Raphson
  cfblk7 : Product
  cfblk8 : Gain  Gain=[364411054.574952]
  cfblk9 : Subsystem
  cfblk2 : Outport
  cfblk12 : Outport  Port=2
  wires:
  cfblk11/1 -> cfblk7/1
  cfblk9/1(cfblk2) -> cfblk6/1
  cfblk10/1 -> cfblk9/1(cfblk1)
  cfblk8/1 -> cfblk9/2(cfblk9)
  cfblk6/1 -> cfblk4/1
  cfblk1/1 -> cfblk7/2
  cfblk3/1 -> cfblk8/1, cfblk12/1
  cfblk7/1 -> cfblk2/1
  cfblk9/2(cfblk11) -> cfblk5/1
  cfblk4/1 -> cfblk13/1
  cfblk13/1 -> cfblk3/1
  cfblk5/1 -> cfblk14/1
  cfblk14/1 -> cfblk9/3(cfblk10)

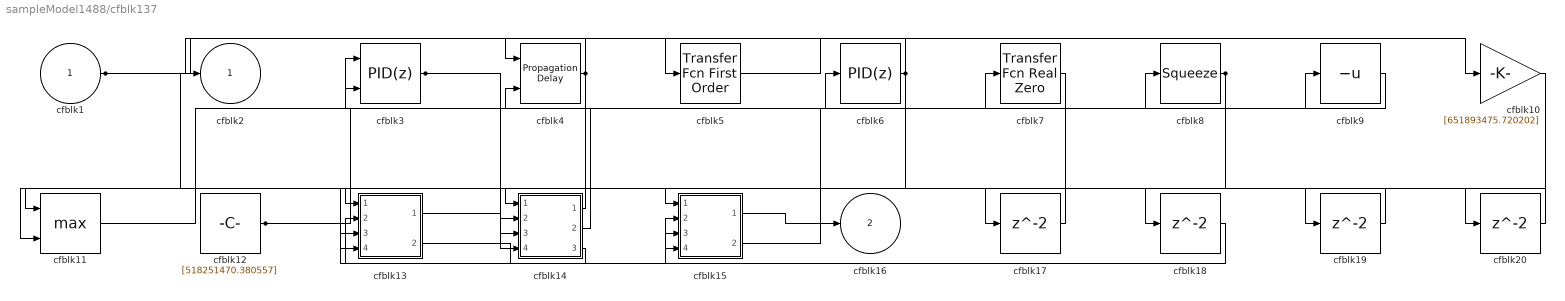
== system sampleModel1488/cfblk137 ==
  cfblk1 : Inport
  cfblk10 : Gain  Gain=[651893475.720202]
  cfblk11 : MinMax  Function=max  Inputs=2
  cfblk12 : Constant  Value=[518251470.380557]  SampleTime=1
  cfblk13 : Subsystem
  cfblk14 : Subsystem
  cfblk15 : Subsystem
  cfblk{17..20} (4 alike) : Delay  SampleTime=1
  cfblk3 : slpidlib/PID Controller (2DOF)  Controller=PID  Form=Parallel  TimeDomain=Discrete-time  UseExternalTs=off  SampleTime=1  IntegratorMethod=Forward Euler  FilterMethod=Forward Euler  ControllerParametersSource=internal  P=1  I=1  UseKiTs=off  D=0  N=100  UseFilter=on  b=1  c=1  TunerSelectOption=Transfer Function Based (PID Tuner App)  InitialConditionSource=internal  InitialConditionForIntegrator=0  InitialConditionForFilter=0  DifferentiatorICPrevScaledInput=0  ExternalReset=none  TrackingMode=off  Kt=1  LimitOutput=off  SatLimitsSource=internal  UpperSaturationLimit=inf  LowerSaturationLimit=-inf  LinearizeAsGain=off  AntiWindupMode=none  Kb=1  LimitIntegrator=off  UpperIntegratorSaturationLimit=inf  LowerIntegratorSaturationLimit=-inf  POutMin=[]  POutMax=[]  IOutMin=[]  IOutMax=[]  DOutMin=[]  DOutMax=[]  NOutMin=[]  NOutMax=[]  bOutMin=[]  bOutMax=[]  cOutMin=[]  cOutMax=[]  SumOutMin=[]  SumOutMax=[]  SaturationOutMin=[]  SaturationOutMax=[]  PParamMin=[]  PParamMax=[]  IParamMin=[]  IParamMax=[]  DParamMin=[]  DParamMax=[]  NParamMin=[]  NParamMax=[]  bParamMin=[]  bParamMax=[]  cParamMin=[]  cParamMax=[]  KbParamMin=[]  KbParamMax=[]  KtParamMin=[]  KtParamMax=[]  KbOutMin=[]  KbOutMax=[]  KtOutMin=[]  KtOutMax=[]  IntegratorOutMin=[]  IntegratorOutMax=[]  FilterOutMin=[]  FilterOutMax=[]  SumI1OutMin=[]  SumI1OutMax=[]  SumI2OutMin=[]  SumI2OutMax=[]  SumI3OutMin=[]  SumI3OutMax=[]  SumI4OutMin=[]  SumI4OutMax=[]  SumDOutMin=[]  SumDOutMax=[]  Sum1OutMin=[]  Sum1OutMax=[]  Sum2OutMin=[]  Sum2OutMax=[]  Sum3OutMin=[]  Sum3OutMax=[]  DifferentiatorOutMin=[]  DifferentiatorOutMax=[]  FilterDiffOutCoefMin=[]  FilterDiffOutCoefMax=[]  ReciprocalOutMin=[]  ReciprocalOutMax=[]  SumDenOutMin=[]  SumDenOutMax=[]  SumNumOutMin=[]  SumNumOutMax=[]  DivideOutMin=[]  DivideOutMax=[]  UdiffTsProdOutMin=[]  UdiffTsProdOutMax=[]  NTsProdOutMin=[]  NTsProdOutMax=[]  UintegralTsProdOutMin=[]  UintegralTsProdOutMax=[]  UngainTsProdOutMin=[]  UngainTsProdOutMax=[]  ClampingZeroOutDataTypeStr=Inherit: Inherit via back propagation  ClampingZeroOutMin=[]  ClampingZeroOutMax=[]  FilterDenConstantOutDataTypeStr=Inherit: Inherit via back propagation  FilterDenConstantOutMin=[]  FilterDenConstantOutMax=[]  PCopyOutDataTypeStr=Inherit: Inherit via back propagation  PCopyOutMin=[]  PCopyOutMax=[]  NCopyOutDataTypeStr=Inherit: Inherit via back propagation  NCopyOutMin=[]  NCopyOutMax=[]  IntegratorContinuousStateAttributes=''  IntegratorStateMustResolveToSignalObject=off  IntegratorRTWStateStorageClass=Auto  FilterContinuousStateAttributes=''  FilterStateMustResolveToSignalObject=off  FilterRTWStateStorageClass=Auto  ParallelPVariant=InternalParameters  IdealPVariant=Disabled  IVariant=InternalParameters  DVariant=InternalParameters  bVariant=InternalParameters  cVariant=InternalParameters  IntegratorVariant=Discrete  SatVariant=Disabled  AWVariant=Passthrough  PCopyVariant=Disabled  TRVariant=Disabled  FdbkBlocksVariant=Forward  IdealPFdbkVariant=Disabled  SatFdbkVariant=Disabled  DerivativeFilterVariant=ForwardEulerFilter  NVariant=InternalParameters  NCopyVariant=Disabled  FilterICVariant=InternalICsFilter  IntegratorICVariant=InternalICs  ExternalResetVariant=Disabled  TRSumVariant=Passthrough  SumFdbkVariant=Disabled  SumVariant=Sum_PID  TsampFilterVariant=InternalTs  TsampNgainVariant=Passthrough  TsampIntegralVariant=Disabled_SignalSpec  ExternalSaturationOutDataTypeStr=Inherit: Same as second input
      settings: LibrarySourceBlock=simulink/Discrete/Discrete PID Controller (2DOF)
  cfblk4 : PropagationDelay  SampleTime=1
  cfblk5 : simulink/Discrete/Transfer Fcn First Order  PoleZ=0.95  ICPrevOutput=0.0  DoSatur=off
  cfblk6 : slpidlib/PID Controller  Controller=PID  Form=Parallel  TimeDomain=Discrete-time  UseExternalTs=off  SampleTime=1  IntegratorMethod=Forward Euler  FilterMethod=Forward Euler  ControllerParametersSource=internal  P=1  I=1  UseKiTs=off  D=0  N=100  UseFilter=on  TunerSelectOption=Transfer Function Based (PID Tuner App)  InitialConditionSource=internal  InitialConditionForIntegrator=0  InitialConditionForFilter=0  DifferentiatorICPrevScaledInput=0  ExternalReset=none  TrackingMode=off  Kt=1  LimitOutput=off  SatLimitsSource=internal  UpperSaturationLimit=inf  LowerSaturationLimit=-inf  LinearizeAsGain=off  AntiWindupMode=none  Kb=1  LimitIntegrator=off  UpperIntegratorSaturationLimit=inf  LowerIntegratorSaturationLimit=-inf  POutMin=[]  POutMax=[]  IOutMin=[]  IOutMax=[]  DOutMin=[]  DOutMax=[]  NOutMin=[]  NOutMax=[]  SumOutMin=[]  SumOutMax=[]  SaturationOutMin=[]  SaturationOutMax=[]  PParamMin=[]  PParamMax=[]  IParamMin=[]  IParamMax=[]  DParamMin=[]  DParamMax=[]  NParamMin=[]  NParamMax=[]  KbParamMin=[]  KbParamMax=[]  KtParamMin=[]  KtParamMax=[]  KbOutMin=[]  KbOutMax=[]  KtOutMin=[]  KtOutMax=[]  IntegratorOutMin=[]  IntegratorOutMax=[]  FilterOutMin=[]  FilterOutMax=[]  SumI1OutMin=[]  SumI1OutMax=[]  SumI2OutMin=[]  SumI2OutMax=[]  SumI3OutMin=[]  SumI3OutMax=[]  SumI4OutMin=[]  SumI4OutMax=[]  SumDOutMin=[]  SumDOutMax=[]  DifferentiatorOutMin=[]  DifferentiatorOutMax=[]  FilterDiffOutCoefMin=[]  FilterDiffOutCoefMax=[]  ReciprocalOutMin=[]  ReciprocalOutMax=[]  SumDenOutMin=[]  SumDenOutMax=[]  SumNumOutMin=[]  SumNumOutMax=[]  DivideOutMin=[]  DivideOutMax=[]  UdiffTsProdOutMin=[]  UdiffTsProdOutMax=[]  NTsProdOutMin=[]  NTsProdOutMax=[]  UintegralTsProdOutMin=[]  UintegralTsProdOutMax=[]  UngainTsProdOutMin=[]  UngainTsProdOutMax=[]  ClampingZeroOutDataTypeStr=Inherit: Inherit via back propagation  ClampingZeroOutMin=[]  ClampingZeroOutMax=[]  FilterDenConstantOutDataTypeStr=Inherit: Inherit via back propagation  FilterDenConstantOutMin=[]  FilterDenConstantOutMax=[]  PCopyOutDataTypeStr=Inherit: Inherit via back propagation  PCopyOutMin=[]  PCopyOutMax=[]  NCopyOutDataTypeStr=Inherit: Inherit via back propagation  NCopyOutMin=[]  NCopyOutMax=[]  IntegratorContinuousStateAttributes=''  IntegratorStateMustResolveToSignalObject=off  IntegratorRTWStateStorageClass=Auto  FilterContinuousStateAttributes=''  FilterStateMustResolveToSignalObject=off  FilterRTWStateStorageClass=Auto  ParallelPVariant=InternalParameters  IdealPVariant=Disabled  IVariant=InternalParameters  DVariant=InternalParameters  IntegratorVariant=Discrete  SatVariant=Disabled  AWVariant=Passthrough  PCopyVariant=Disabled  TRVariant=Disabled  FdbkBlocksVariant=Forward  IdealPFdbkVariant=Disabled  SatFdbkVariant=Disabled  DerivativeFilterVariant=ForwardEulerFilter  NVariant=InternalParameters  NCopyVariant=Disabled  FilterICVariant=InternalICsFilter  IntegratorICVariant=InternalICs  ExternalResetVariant=Disabled  TRSumVariant=Passthrough  SumFdbkVariant=Disabled  SumVariant=Sum_PID  TsampFilterVariant=InternalTs  TsampNgainVariant=Passthrough  TsampIntegralVariant=Disabled_SignalSpec  ExternalSaturationOutDataTypeStr=Inherit: Same as second input
      settings: LibrarySourceBlock=simulink/Discrete/Discrete PID Controller
  cfblk7 : simulink/Discrete/Transfer Fcn Real Zero  ZeroZ=0.75  ICPrevInput=0.0  DoSatur=off
  cfblk8 : Squeeze
  cfblk9 : UnaryMinus
  cfblk2 : Outport
  cfblk16 : Outport  Port=2
  wires:
  cfblk11/1 -> cfblk7/1
  cfblk12/1 -> cfblk6/1, cfblk15/3(cfblk9)
  cfblk14/1(cfblk2) -> cfblk3/1
  cfblk6/1 -> cfblk4/1, cfblk14/4(cfblk12), cfblk13/3(cfblk11), cfblk13/4(cfblk12)
  cfblk5/1 -> cfblk10/1
  cfblk3/1 -> cfblk19/1, cfblk20/1
  cfblk9/1 -> cfblk8/1
  cfblk8/1 -> cfblk4/2, cfblk18/1
  cfblk1/1 -> cfblk5/1, cfblk14/3(cfblk11)
  cfblk15/1(cfblk2) -> cfblk16/1
  cfblk15/2(cfblk11) -> cfblk9/1
  cfblk14/2(cfblk13) -> cfblk3/2
  cfblk10/1 -> cfblk13/1(cfblk1)
  cfblk4/1 -> cfblk11/2, cfblk2/1
  cfblk14/3(cfblk14) -> cfblk13/2(cfblk10)
  cfblk13/1(cfblk2) -> cfblk15/1(cfblk1)
  cfblk13/2(cfblk13) -> cfblk15/2(cfblk8)
  cfblk7/1 -> cfblk17/1
  cfblk17/1 -> cfblk11/1
  cfblk18/1 -> cfblk15/4(cfblk10)
  cfblk19/1 -> cfblk14/1(cfblk1)
  cfblk20/1 -> cfblk14/2(cfblk10)

== system sampleModel1488/cfblk138 ==
  cfblk1 : Inport
  cfblk9 : Inport  Port=2
  cfblk3 : DiscreteTransferFcn  SampleTime=1
  cfblk4 : DiscreteZeroPole  Poles=[0 0.5]  Gain=1
  cfblk5 : slpidlib/PID Controller  Controller=PID  Form=Parallel  TimeDomain=Discrete-time  UseExternalTs=off  SampleTime=1  IntegratorMethod=Forward Euler  FilterMethod=Forward Euler  ControllerParametersSource=internal  P=1  I=1  UseKiTs=off  D=0  N=100  UseFilter=on  TunerSelectOption=Transfer Function Based (PID Tuner App)  InitialConditionSource=internal  InitialConditionForIntegrator=0  InitialConditionForFilter=0  DifferentiatorICPrevScaledInput=0  ExternalReset=none  TrackingMode=off  Kt=1  LimitOutput=off  SatLimitsSource=internal  UpperSaturationLimit=inf  LowerSaturationLimit=-inf  LinearizeAsGain=off  AntiWindupMode=none  Kb=1  LimitIntegrator=off  UpperIntegratorSaturationLimit=inf  LowerIntegratorSaturationLimit=-inf  POutMin=[]  POutMax=[]  IOutMin=[]  IOutMax=[]  DOutMin=[]  DOutMax=[]  NOutMin=[]  NOutMax=[]  SumOutMin=[]  SumOutMax=[]  SaturationOutMin=[]  SaturationOutMax=[]  PParamMin=[]  PParamMax=[]  IParamMin=[]  IParamMax=[]  DParamMin=[]  DParamMax=[]  NParamMin=[]  NParamMax=[]  KbParamMin=[]  KbParamMax=[]  KtParamMin=[]  KtParamMax=[]  KbOutMin=[]  KbOutMax=[]  KtOutMin=[]  KtOutMax=[]  IntegratorOutMin=[]  IntegratorOutMax=[]  FilterOutMin=[]  FilterOutMax=[]  SumI1OutMin=[]  SumI1OutMax=[]  SumI2OutMin=[]  SumI2OutMax=[]  SumI3OutMin=[]  SumI3OutMax=[]  SumI4OutMin=[]  SumI4OutMax=[]  SumDOutMin=[]  SumDOutMax=[]  DifferentiatorOutMin=[]  DifferentiatorOutMax=[]  FilterDiffOutCoefMin=[]  FilterDiffOutCoefMax=[]  ReciprocalOutMin=[]  ReciprocalOutMax=[]  SumDenOutMin=[]  SumDenOutMax=[]  SumNumOutMin=[]  SumNumOutMax=[]  DivideOutMin=[]  DivideOutMax=[]  UdiffTsProdOutMin=[]  UdiffTsProdOutMax=[]  NTsProdOutMin=[]  NTsProdOutMax=[]  UintegralTsProdOutMin=[]  UintegralTsProdOutMax=[]  UngainTsProdOutMin=[]  UngainTsProdOutMax=[]  ClampingZeroOutDataTypeStr=Inherit: Inherit via back propagation  ClampingZeroOutMin=[]  ClampingZeroOutMax=[]  FilterDenConstantOutDataTypeStr=Inherit: Inherit via back propagation  FilterDenConstantOutMin=[]  FilterDenConstantOutMax=[]  PCopyOutDataTypeStr=Inherit: Inherit via back propagation  PCopyOutMin=[]  PCopyOutMax=[]  NCopyOutDataTypeStr=Inherit: Inherit via back propagation  NCopyOutMin=[]  NCopyOutMax=[]  IntegratorContinuousStateAttributes=''  IntegratorStateMustResolveToSignalObject=off  IntegratorRTWStateStorageClass=Auto  FilterContinuousStateAttributes=''  FilterStateMustResolveToSignalObject=off  FilterRTWStateStorageClass=Auto  ParallelPVariant=InternalParameters  IdealPVariant=Disabled  IVariant=InternalParameters  DVariant=InternalParameters  IntegratorVariant=Discrete  SatVariant=Disabled  AWVariant=Passthrough  PCopyVariant=Disabled  TRVariant=Disabled  FdbkBlocksVariant=Forward  IdealPFdbkVariant=Disabled  SatFdbkVariant=Disabled  DerivativeFilterVariant=ForwardEulerFilter  NVariant=InternalParameters  NCopyVariant=Disabled  FilterICVariant=InternalICsFilter  IntegratorICVariant=InternalICs  ExternalResetVariant=Disabled  TRSumVariant=Passthrough  SumFdbkVariant=Disabled  SumVariant=Sum_PID  TsampFilterVariant=InternalTs  TsampNgainVariant=Passthrough  TsampIntegralVariant=Disabled_SignalSpec  ExternalSaturationOutDataTypeStr=Inherit: Same as second input
      settings: LibrarySourceBlock=simulink/Discrete/Discrete PID Controller
  cfblk6 : Reshape
  cfblk7 : Subsystem
  cfblk8 : Subsystem
  cfblk2 : Outport
  cfblk10 : Outport  Port=2
  wires:
  cfblk1/1 -> cfblk5/1
  cfblk5/1 -> cfblk8/1(cfblk1)
  cfblk4/1 -> cfblk10/1
  cfblk7/1(cfblk2) -> cfblk6/1
  cfblk7/2(cfblk7) -> cfblk3/1
  cfblk9/1 -> cfblk7/1(cfblk1), cfblk8/2(cfblk9)
  cfblk6/1 -> cfblk4/1
  cfblk3/1 -> cfblk2/1
  cfblk8/1(cfblk2) -> cfblk7/2(cfblk5)
  cfblk8/2(cfblk10) -> cfblk7/3(cfblk6)

== system sampleModel1488/cfblk139 ==
  cfblk1 : Inport
  cfblk10 : Subsystem
  cfblk11 : Subsystem
  cfblk12 : Subsystem
  cfblk{14..18} (5 alike) : Delay  SampleTime=1
  cfblk3 : DiscreteTransferFcn  SampleTime=1
  cfblk4 : simulink/Math Operations/Slider Gain  gain=1  low=0  high=2
  cfblk5 : Sqrt
  cfblk6 : Squeeze
  cfblk7 : Constant  Value=[-595999081.343417]  SampleTime=1
  cfblk8 : Subsystem
  cfblk9 : Subsystem
  cfblk2 : Outport
  cfblk13 : Outport  Port=2
  wires:
  cfblk3/1 -> cfblk2/1, cfblk9/4(cfblk15)
  cfblk5/1 -> cfblk13/1
  cfblk10/1(cfblk2) -> cfblk11/1(cfblk1)
  cfblk11/1(cfblk2) -> cfblk9/1(cfblk1)
  cfblk12/1(cfblk2) -> cfblk10/1(cfblk1), cfblk8/2(cfblk5), cfblk9/2(cfblk13)
  cfblk4/1 -> cfblk5/1, cfblk8/1(cfblk1)
  cfblk8/1(cfblk2) -> cfblk3/1
  cfblk11/2(cfblk10) -> cfblk6/1
  cfblk8/3(cfblk7) -> cfblk9/3(cfblk14), cfblk18/1
  cfblk7/1 -> cfblk12/1(cfblk1), cfblk12/5(cfblk10)
  cfblk6/1 -> cfblk4/1, cfblk16/1
  cfblk1/1 -> cfblk12/4(cfblk9), cfblk11/4(cfblk9)
  cfblk9/1(cfblk2) -> cfblk14/1
  cfblk14/1 -> cfblk11/3(cfblk8)
  cfblk9/2(cfblk16) -> cfblk15/1
  cfblk15/1 -> cfblk12/2(cfblk7)
  cfblk16/1 -> cfblk12/3(cfblk8)
  cfblk8/2(cfblk6) -> cfblk17/1
  cfblk17/1 -> cfblk11/2(cfblk7)
  cfblk18/1 -> cfblk10/2(cfblk8)
